simulink model "PIDcontrol"  (R2020b)
settings: Solver=VariableStepAuto  StartTime=0.0  StopTime=500  RelTol=1e-3
libraries: pid_lib x1
settings Model: Creator=orangejuzi  LastModifiedBy=orangejuzi
settings SolverCC: MaxConsecutiveZCs=1  ZeroCrossAlgorithm=Adaptive
settings DebuggingCC: IgnoredZcDiagnostic=none

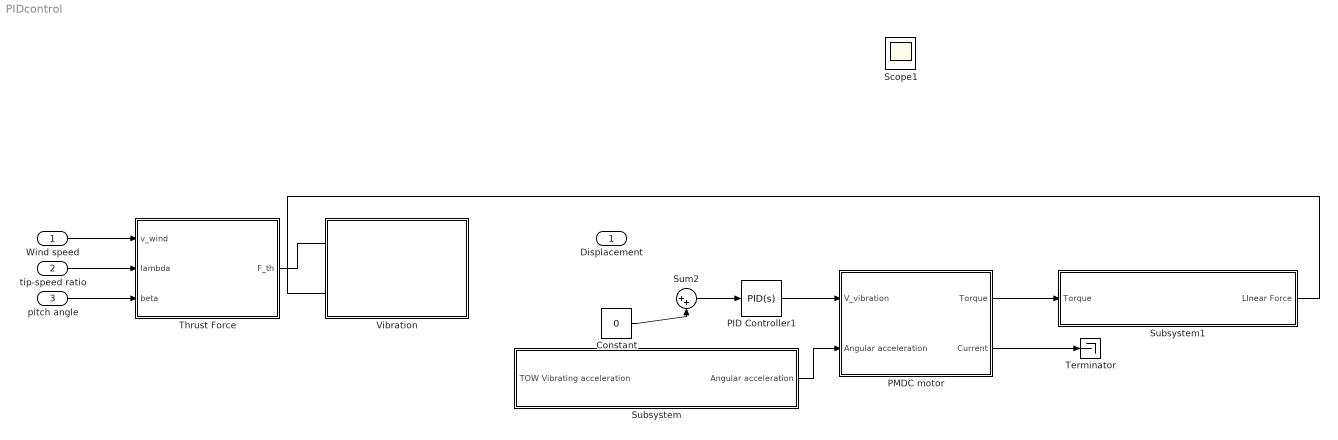
== system PIDcontrol ==
  Wind speed : Inport
  tip-speed ratio : Inport  Port=2
  "pitch angle " : Inport  Port=3
  Constant : Constant  Value=0
  PID Controller1 : pid_lib/PID Controller  Controller=PID  Form=Parallel  TimeDomain=Continuous-time  UseExternalTs=off  SampleTime=-1  IntegratorMethod=Forward Euler  FilterMethod=Forward Euler  ControllerParametersSource=internal  P=1  I=1  D=0  UseFilter=on  N=100  TunerSelectOption=Transfer Function Based (PID Tuner App)  InitialConditionSource=internal  InitialConditionForIntegrator=0  InitialConditionForFilter=0  DifferentiatorICPrevScaledInput=0  ExternalReset=none  TrackingMode=off  Kt=1  LimitOutput=off  SatLimitsSource=internal  UpperSaturationLimit=inf  LowerSaturationLimit=-inf  LinearizeAsGain=on  AntiWindupMode=none  Kb=1  POutMin=[]  POutMax=[]  IOutMin=[]  IOutMax=[]  DOutMin=[]  DOutMax=[]  NOutMin=[]  NOutMax=[]  SumOutMin=[]  SumOutMax=[]  SaturationOutMin=[]  SaturationOutMax=[]  PParamMin=[]  PParamMax=[]  IParamMin=[]  IParamMax=[]  DParamMin=[]  DParamMax=[]  NParamMin=[]  NParamMax=[]  KbParamMin=[]  KbParamMax=[]  KtParamMin=[]  KtParamMax=[]  KbOutMin=[]  KbOutMax=[]  KtOutMin=[]  KtOutMax=[]  IntegratorOutMin=[]  IntegratorOutMax=[]  FilterOutMin=[]  FilterOutMax=[]  SumI1OutMin=[]  SumI1OutMax=[]  SumI2OutMin=[]  SumI2OutMax=[]  SumI3OutMin=[]  SumI3OutMax=[]  SumI4OutMin=[]  SumI4OutMax=[]  SumDOutMin=[]  SumDOutMax=[]  DifferentiatorOutMin=[]  DifferentiatorOutMax=[]  FilterDiffOutCoefMin=[]  FilterDiffOutCoefMax=[]  ReciprocalOutMin=[]  ReciprocalOutMax=[]  SumDenOutMin=[]  SumDenOutMax=[]  SumNumOutMin=[]  SumNumOutMax=[]  DivideOutMin=[]  DivideOutMax=[]  UdiffTsProdOutMin=[]  UdiffTsProdOutMax=[]  NTsProdOutMin=[]  NTsProdOutMax=[]  UintegralTsProdOutMin=[]  UintegralTsProdOutMax=[]  UngainTsProdOutMin=[]  UngainTsProdOutMax=[]  IntegratorContinuousStateAttributes=''  IntegratorStateMustResolveToSignalObject=off  IntegratorRTWStateStorageClass=Auto  FilterContinuousStateAttributes=''  FilterStateMustResolveToSignalObject=off  FilterRTWStateStorageClass=Auto  ParallelPVariant=InternalParameters  IdealPVariant=Disabled  IVariant=InternalParameters  DVariant=InternalParameters  IntegratorVariant=Continuous  SatVariant=Disabled  AWVariant=Passthrough  PCopyVariant=Disabled  TRVariant=Disabled  FdbkBlocksVariant=Forward  IdealPFdbkVariant=Disabled  SatFdbkVariant=Disabled  DerivativeFilterVariant=ContFilter  NVariant=InternalParameters  NCopyVariant=Disabled  FilterICVariant=InternalICsFilter  IntegratorICVariant=InternalICs  ExternalResetVariant=Disabled  TRSumVariant=Passthrough  SumFdbkVariant=Disabled  SumVariant=Sum_PID  TsampFilterVariant=InternalTs  TsampNgainVariant=Passthrough  TsampIntegralVariant=Passthrough  ExternalSaturationOutDataTypeStr=Inherit: Same as second input
  PMDC motor : Subsystem
  Scope1 : Scope
  Subsystem : Subsystem
  Subsystem1 : Subsystem
  Sum2 : Sum  Inputs=|++
  Terminator : Terminator
  Thrust Force : Subsystem
  Vibration : Subsystem
  Displacement : Outport
  wires:
  Sum2/1 -> PID Controller1/1
  PID Controller1/1 -> PMDC motor/1(V_vibration)
  ? -> Subsystem/1(TOW Vibrating acceleration)
  Subsystem1/1(LInear Force) -> ?
  Constant/1 -> Sum2/2
  Thrust Force/1(F_th) -> ?
  Subsystem/1(Angular acceleration) -> PMDC motor/2(Angular acceleration)
  Wind speed/1 -> Thrust Force/1(v_wind)
  "pitch angle "/1 -> Thrust Force/3(beta)
  tip-speed ratio/1 -> Thrust Force/2(lambda)
  ? -> Sum2/1
  PMDC motor/2(Current) -> Terminator/1
  ? -> Displacement/1
  PMDC motor/1(Torque) -> Subsystem1/1(Torque)

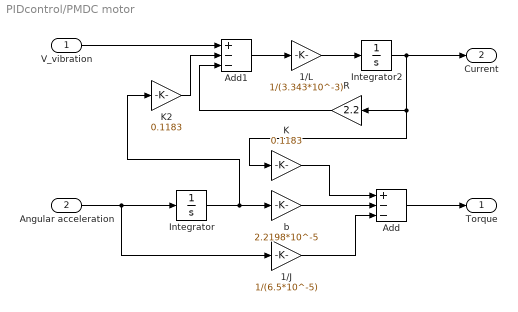
== system PIDcontrol/PMDC motor ==
  V_vibration : Inport
  Angular acceleration : Inport  Port=2
  1/J : Gain  Gain=1/(6.5*10^-5)
  1/L : Gain  Gain=1/(3.343*10^-3)
  Add : Sum  Inputs=+--
  Add1 : Sum  Inputs=+--
  Integrator : Integrator
  Integrator2 : Integrator
  K : Gain  Gain=0.1183
  K2 : Gain  Gain=0.1183
  R : Gain  Gain=2.2
  b : Gain  Gain=2.2198*10^-5
  Torque : Outport
  Current : Outport  Port=2
  wires:
  Add/1 -> Torque/1
  K2/1 -> Add1/2
  Integrator2/1 -> R/1, K/1, Current/1
  1/L/1 -> Integrator2/1
  Add1/1 -> 1/L/1
  K/1 -> Add/1
  R/1 -> Add1/3
  V_vibration/1 -> Add1/1
  Angular acceleration/1 -> 1/J/1, Integrator/1
  Integrator/1 -> K2/1, b/1
  b/1 -> Add/2
  1/J/1 -> Add/3

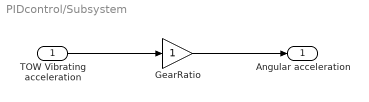
== system PIDcontrol/Subsystem ==
  TOW Vibrating acceleration : Inport
  GearRatio : Gain
  Angular acceleration : Outport
  wires:
  TOW Vibrating acceleration/1 -> GearRatio/1
  GearRatio/1 -> Angular acceleration/1

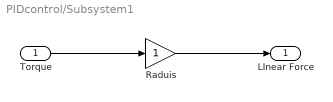
== system PIDcontrol/Subsystem1 ==
  Torque : Inport
  Raduis : Gain
  LInear Force : Outport
  wires:
  Torque/1 -> Raduis/1
  Raduis/1 -> LInear Force/1

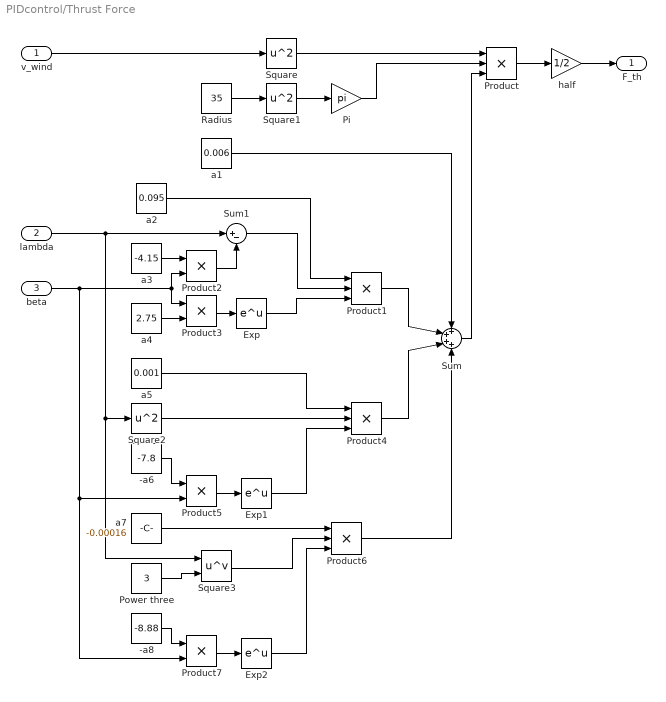
== system PIDcontrol/Thrust Force ==
  v_wind : Inport
  lambda : Inport  Port=2
  beta : Inport  Port=3
  -a6 : Constant  Value=-7.8
  -a8 : Constant  Value=-8.88
  Exp : Math  SaturateOnIntegerOverflow=on
  Exp1 : Math  SaturateOnIntegerOverflow=on
  Exp2 : Math  SaturateOnIntegerOverflow=on
  Pi : Gain  Gain=pi
  Power three : Constant  Value=3
  Product{,1,4,6} (4 alike) : Product  Inputs=3
  Product{2..3,5,7} (4 alike) : Product
  Radius : Constant  Value=35
  Square : Math  Operator=square  SaturateOnIntegerOverflow=on
  Square1 : Math  Operator=square  SaturateOnIntegerOverflow=on
  Square2 : Math  Operator=square  SaturateOnIntegerOverflow=on
  Square3 : Math  Operator=pow  SaturateOnIntegerOverflow=on
  Sum : Sum  Inputs=4
  Sum1 : Sum  Inputs=|+-
  a1 : Constant  Value=0.006
  a2 : Constant  Value=0.095
  a3 : Constant  Value=-4.15
  a4 : Constant  Value=2.75
  a5 : Constant  Value=0.001
  a7 : Constant  Value=-0.00016
  half : Gain  Gain=1/2
  F_th : Outport
  wires:
  v_wind/1 -> Square/1
  half/1 -> F_th/1
  Product/1 -> half/1
  Square/1 -> Product/1
  Radius/1 -> Square1/1
  Square1/1 -> Pi/1
  Pi/1 -> Product/2
  Sum/1 -> Product/3
  a1/1 -> Sum/1
  a2/1 -> Product1/1
  Sum1/1 -> Product1/2
  lambda/1 -> Sum1/1, Square2/1, Square3/1
  Product2/1 -> Sum1/2
  a3/1 -> Product2/1
  beta/1 -> Product3/1, Product2/2, Product5/2, Product7/2
  Exp/1 -> Product1/3
  Product3/1 -> Exp/1
  a4/1 -> Product3/2
  Product1/1 -> Sum/2
  -a6/1 -> Product5/1
  Product5/1 -> Exp1/1
  Exp1/1 -> Product4/3
  Square2/1 -> Product4/2
  a5/1 -> Product4/1
  Product4/1 -> Sum/3
  Exp2/1 -> Product6/3
  Square3/1 -> Product6/2
  a7/1 -> Product6/1
  -a8/1 -> Product7/1
  Product7/1 -> Exp2/1
  Power three/1 -> Square3/2
  Product6/1 -> Sum/4

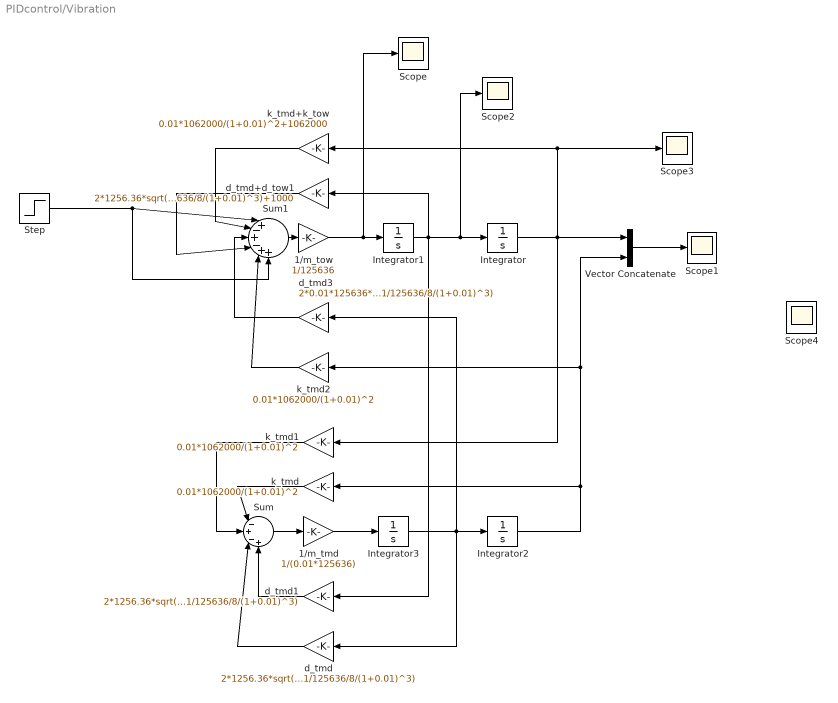
== system PIDcontrol/Vibration ==
  1/m_tmd : Gain  Gain=1/(0.01*125636)
  1/m_tow : Gain  Gain=1/125636
  Integrator{,1..3} (4 alike) : Integrator
  Scope{,1..4} (5 alike) : Scope
  Step : Step  SampleTime=0
  Sum : Sum  Inputs=|-+-+
  Sum1 : Sum  Inputs=|+-+-++
  Vector Concatenate : Concatenate
  d_tmd : Gain  Gain=2*1256.36*sqrt(1062000/125636)*sqrt(1062000*3*0.01/125636/8/(1+0.01)^3)
  d_tmd+d_tow1 : Gain  Gain=2*1256.36*sqrt(1062000/125636)*sqrt(1062000*3*0.01/125636/8/(1+0.01)^3)+1000
  d_tmd1 : Gain  Gain=2*1256.36*sqrt(1062000/125636)*sqrt(1062000*3*0.01/125636/8/(1+0.01)^3)
  d_tmd3 : Gain  Gain=2*0.01*125636*sqrt(1062000*3*0.01/125636/8/(1+0.01)^3)
  k_tmd : Gain  Gain=0.01*1062000/(1+0.01)^2
  k_tmd+k_tow : Gain  Gain=0.01*1062000/(1+0.01)^2+1062000
  k_tmd1 : Gain  Gain=0.01*1062000/(1+0.01)^2
  k_tmd2 : Gain  Gain=0.01*1062000/(1+0.01)^2
  wires:
  Integrator1/1 -> d_tmd+d_tow1/1, d_tmd1/1, Scope2/1, Integrator/1
  Integrator/1 -> Scope3/1, k_tmd+k_tow/1, Vector Concatenate/1, k_tmd1/1
  Integrator3/1 -> d_tmd/1, d_tmd3/1, Integrator2/1
  1/m_tmd/1 -> Integrator3/1
  Sum/1 -> 1/m_tmd/1
  1/m_tow/1 -> Scope/1, Integrator1/1
  Sum1/1 -> 1/m_tow/1
  k_tmd/1 -> Sum/1
  d_tmd/1 -> Sum/3
  d_tmd1/1 -> Sum/4
  k_tmd1/1 -> Sum/2
  k_tmd+k_tow/1 -> Sum1/2
  d_tmd+d_tow1/1 -> Sum1/4
  d_tmd3/1 -> Sum1/3
  Integrator2/1 -> k_tmd/1, k_tmd2/1, Vector Concatenate/2
  k_tmd2/1 -> Sum1/5
  Vector Concatenate/1 -> Scope1/1
  Step/1 -> Sum1/1, Sum1/6
